simulink model "Linear_Model"  (R2021a)
settings: Solver=VariableStepAuto  StartTime=0.0  StopTime=20  RelTol=1e-3
values from neighbouring files (symbols this model uses):
  A = [ a11,a12,a13 ... (first row only)    [Linearmodel.m]    (also in matlab.mat = [-1  1; 0  1])
  B = [ b11,b12 ... (first row only)    [Linearmodel.m]    (also in matlab.mat = [0 1])
  C = eye(9)    [Linearmodel.m]    (also in matlab.mat = [1 0])
  D = zeros(9,4)    [Linearmodel.m]    (also in matlab.mat = 0)
  K = lqr(A,B,Q,R)    [Linearmodel.m]    (also in matlab.mat = [20 20])
  Ki = lqr(Ai,Bi,Qi,Ri)    [Linearmodel.m]
  x0 = [1,0,0,0,0,0,0,0,0]'    [Linearmodel.m]
settings Model: Creator=Sirius  LastModifiedBy=Sirius

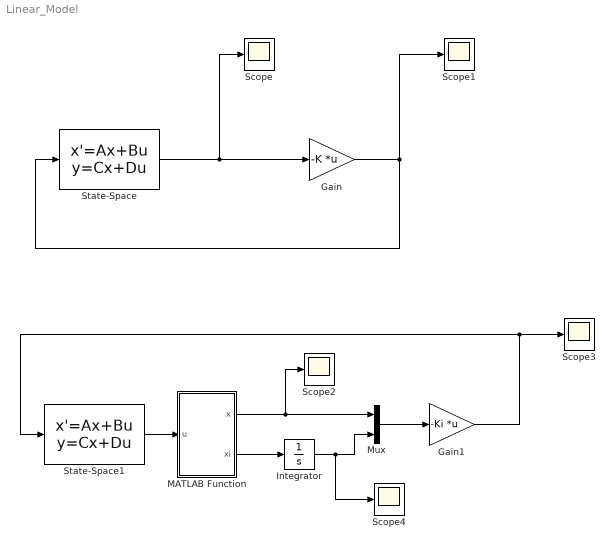
== system Linear_Model ==
  Gain : Gain  Gain=-K  Multiplication=Matrix(K*u)
  Gain1 : Gain  Gain=-Ki  Multiplication=Matrix(K*u)
  Integrator : Integrator  InitialCondition=[0;0;0;0]
  MATLAB Function : MATLAB Function  TreatAsAtomicUnit=on
  Mux : Mux  Inputs=2
  Scope{,1..4} (5 alike) : Scope
  State-Space : StateSpace  A=A  B=B  C=C  D=D  InitialCondition=x0
  State-Space1 : StateSpace  A=A  B=B  C=C  D=D  InitialCondition=x0
  wires:
  State-Space/1 -> Scope/1, Gain/1
  Gain/1 -> State-Space/1, Scope1/1
  Gain1/1 -> State-Space1/1, Scope3/1
  State-Space1/1 -> MATLAB Function/1(u)
  MATLAB Function/2(xi) -> Integrator/1
  MATLAB Function/1(x) -> Scope2/1, Mux/1
  Integrator/1 -> Scope4/1, Mux/2
  Mux/1 -> Gain1/1

== matlab function Linear_Model/MATLAB Function ==
  data: u input; x output; xi output
function [x,xi] = fcn(u)
x=u(1:9);
xi=[u(1:3);u(9)];
end
